simulink model "three_phase_contactor"  (R2017b)
settings: Solver=VariableStepAuto  StartTime=0.0  StopTime=10.0  RelTol=1e-3
undefined symbols (not defined in the file): S2
libraries: powerlib x5, typhoonHILlib x1
settings Model: Creator=Marcos  LastModifiedBy=Marcos

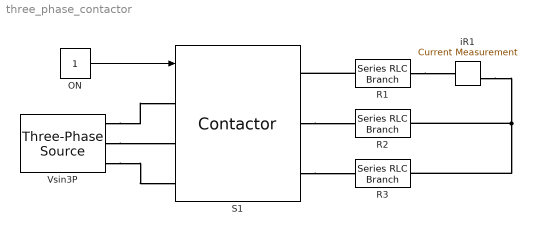
== system three_phase_contactor ==
  ON : Constant
  R1 : powerlib/Elements/Series RLC Branch  LConnTagsString=__new0  RConnTagsString=__new0  BranchType=R  Resistance=10  Inductance=1e-3  SetiL0=off  InitialCurrent=0  Capacitance=1e-6  Setx0=off  InitialVoltage=0  Measurements=None
  R2 : powerlib/Elements/Series RLC Branch  LConnTagsString=__new0  RConnTagsString=__new0  BranchType=R  Resistance=10  Inductance=1e-3  SetiL0=off  InitialCurrent=0  Capacitance=1e-6  Setx0=off  InitialVoltage=0  Measurements=None
  R3 : powerlib/Elements/Series RLC Branch  LConnTagsString=__new0  RConnTagsString=__new0  BranchType=R  Resistance=10  Inductance=1e-3  SetiL0=off  InitialCurrent=0  Capacitance=1e-6  Setx0=off  InitialVoltage=0  Measurements=None
  S1 : typhoonHILlib/Contactor  ContType=Triple Pole Single Throw  init_state=Off / S2  s1_logic=Active-high  di_1=1  tr1_delay=0  tr2_delay=0  r_on=0.001  v_f=0  r_s=1e4  c_s=inf  s0=0  toggle_init=on  old_pat=typhoonPatterns/TPST Contactor  old_size=125,156  model_loaded=off
      settings: SourceProductName=Typhoon HIL
  Vsin3P : powerlib/Electrical Sources/Three-Phase Source  InternalConnection=Yg  VoltagePhases=off  Voltage=381  PhaseAngle=0  Voltage_phases=[25e3 25e3 25e3]/sqrt(3)  PhaseAngles_phases=[0 -120 +120]  Frequency=50  NonIdealSource=off  SpecifyImpedance=off  Resistance=0.8929  Inductance=16.58e-3  ShortCircuitLevel=100e6  BaseVoltage=25e3  XRratio=7  BusType=swing  Pref=10e3  Qref=0  Prefabc=[10e3, 10e3, 10e3]  Qrefabc=[0, 0, 0]  Qmin=-inf  Qmax=inf
  iR1 : powerlib/Measurements/Current Measurement  PhasorSimulation=off  OutputType=Complex  PSBequivalent=0
  wires:
  ON/1 -> S1/1
  connections:
  iR1/RConn1 -- R3/RConn1 -- R2/RConn1
  R1/RConn1 -- iR1/LConn1
  S1/RConn3 -- R3/LConn1
  S1/RConn2 -- R2/LConn1
  R1/LConn1 -- S1/RConn1
  Vsin3P/RConn1 -- S1/LConn1
  Vsin3P/RConn3 -- S1/LConn3
  Vsin3P/RConn2 -- S1/LConn2
